simulink model "discrete_system"  (R2022a)
settings: Solver=FixedStepDiscrete  StartTime=0.0  StopTime=10  FixedStep=2E-4
values from neighbouring files (symbols this model uses):
  a1 = -z2/z1    (= 0.769230769231)    [params.m]    (also in params_nolinear_system.m = -z2/z1)
  a2 = z2*eps/z1    (= 2.331002331)    [params.m]    (also in params_nolinear_system.m = z2*eps/z1)
  a3 = z3/z1    (= 2.47815294211)    [params.m]    (also in params_nolinear_system.m = z3/z1)
  a4 = k/z1    (= 1.09686889935)    [params.m]    (also in params_nolinear_system.m = k/z1)
  b1 = -z4/z5    (= 0.822324878959)    [params.m]    (also in params_nolinear_system.m = -z4/z5)
  b2 = z7/(eps*z5)    (= 8.06700706259)    [params.m]    (also in params_nolinear_system.m = z7/(eps*z5))
  b3 = z6/z5    (= 0.963345768584)    [params.m]    (also in params_nolinear_system.m = z6/z5)
  b4 = -k/z5    (= 0.426391767402)    [params.m]    (also in params_nolinear_system.m = -k/z5)
  K = [1 1 1 1]    [params.m]
undefined symbols (not defined in the file or in its folder): DiscIntNeverNeededParam, magnitude
libraries: simulink x2
settings Model: Creator=epyur  LastModifiedBy=epyur
settings SolverCC: ZeroCrossControl=DisableAll  ZeroCrossAlgorithm=Adaptive

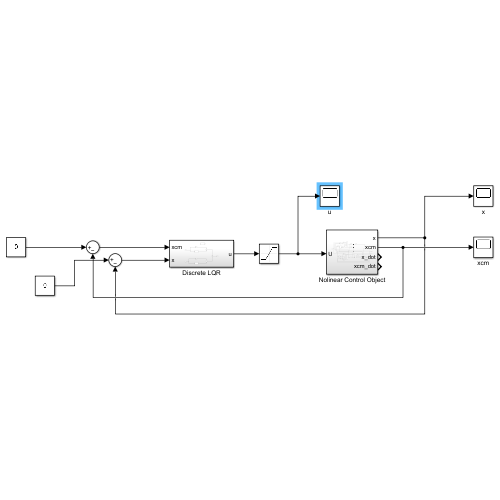
[thumbnail: Simulink's stored preview of the top-level diagram]
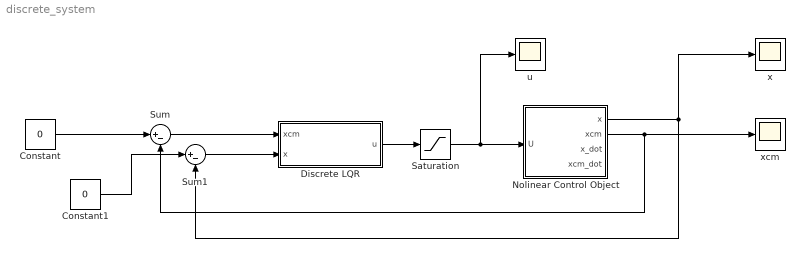
== system discrete_system ==
  Constant : Constant  Value=0
  Constant1 : Constant  Value=0
  Discrete LQR : Subsystem
  Nolinear Control Object : Subsystem
  Saturation : Saturate  UpperLimit=24  LowerLimit=-24
  Sum : Sum  Inputs=|+-
  Sum1 : Sum  Inputs=|+-
  u : Scope
  x : Scope
  xcm : Scope
  wires:
  Saturation/1 -> Nolinear Control Object/1(U), u/1
  Nolinear Control Object/2(xcm) -> Sum/2, xcm/1
  Nolinear Control Object/1(x) -> x/1, Sum1/2
  Discrete LQR/1(u) -> Saturation/1
  Sum/1 -> Discrete LQR/1(xcm)
  Sum1/1 -> Discrete LQR/2(x)
  Constant/1 -> Sum/1
  Constant1/1 -> Sum1/1

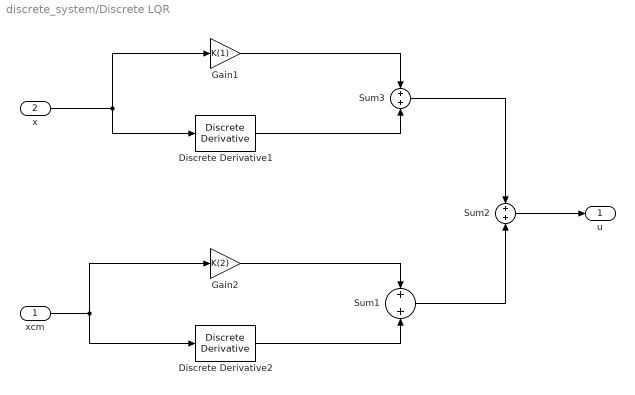
== system discrete_system/Discrete LQR ==
  xcm : Inport
  x : Inport  Port=2
  Discrete Derivative1 : simulink/Discrete/Discrete Derivative  gainval=K(3)  ICPrevScaledInput=0.0  OutMin=[]  OutMax=[]  OutDataType=fixdt(1, 16)  OutScaling=2^-10  DoSatur=off
  Discrete Derivative2 : simulink/Discrete/Discrete Derivative  gainval=K(4)  ICPrevScaledInput=0.0  OutMin=[]  OutMax=[]  OutDataType=fixdt(1, 16)  OutScaling=2^-10  DoSatur=off
  Gain1 : Gain  Gain=K(1)
  Gain2 : Gain  Gain=K(2)
  Sum1 : Sum  Inputs=+|+
  Sum2 : Sum  Inputs=+|+
  Sum3 : Sum  Inputs=+|+
  u : Outport
  wires:
  Sum1/1 -> Sum2/2
  Sum3/1 -> Sum2/1
  Sum2/1 -> u/1
  x/1 -> Discrete Derivative1/1, Gain1/1
  xcm/1 -> Gain2/1, Discrete Derivative2/1
  Discrete Derivative1/1 -> Sum3/2
  Gain1/1 -> Sum3/1
  Discrete Derivative2/1 -> Sum1/2
  Gain2/1 -> Sum1/1

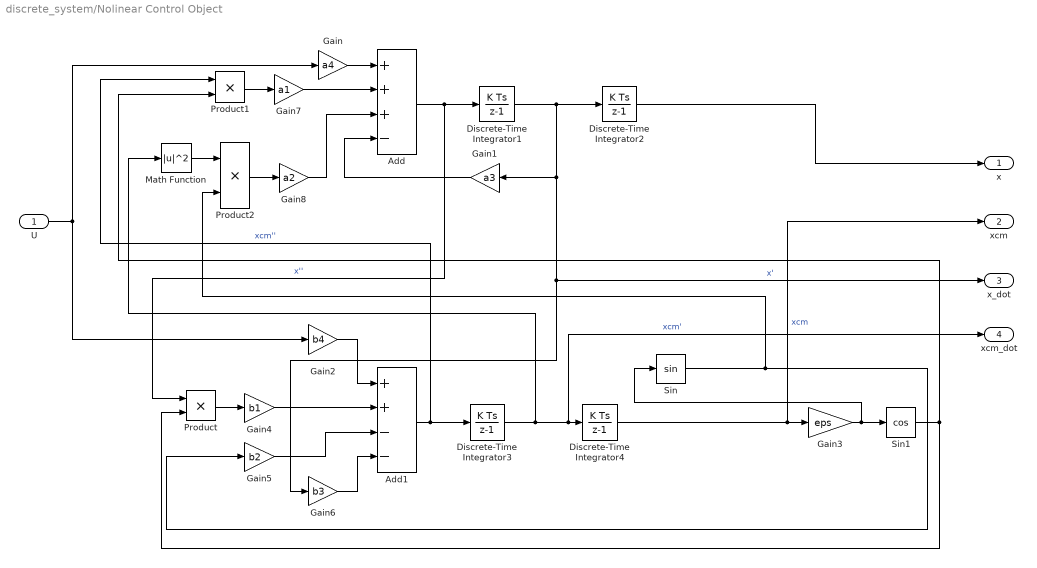
== system discrete_system/Nolinear Control Object ==
  U : Inport
  Add : Sum  Inputs=+++-
  Add1 : Sum  Inputs=++--
  Discrete-Time Integrator1 : DiscreteIntegrator  SampleTime=2e-4  ICPrevOutput=DiscIntNeverNeededParam  ICPrevScaledInput=DiscIntNeverNeededParam
  Discrete-Time Integrator2 : DiscreteIntegrator  SampleTime=2e-4  ICPrevOutput=DiscIntNeverNeededParam  ICPrevScaledInput=DiscIntNeverNeededParam
  Discrete-Time Integrator3 : DiscreteIntegrator  SampleTime=2e-4  ICPrevOutput=DiscIntNeverNeededParam  ICPrevScaledInput=DiscIntNeverNeededParam
  Discrete-Time Integrator4 : DiscreteIntegrator  InitialCondition=-0.144  SampleTime=2e-4  ICPrevOutput=DiscIntNeverNeededParam  ICPrevScaledInput=DiscIntNeverNeededParam
  Gain : Gain  Gain=a4
  Gain1 : Gain  Gain=a3
  Gain2 : Gain  Gain=b4
  Gain3 : Gain  Gain=eps
  Gain4 : Gain  Gain=b1
  Gain5 : Gain  Gain=b2
  Gain6 : Gain  Gain=b3
  Gain7 : Gain  Gain=a1
  Gain8 : Gain  Gain=a2
  Math Function : Math  Operator=magnitude^2
  Product : Product
  Product1 : Product
  Product2 : Product
  Sin : Trigonometry
  Sin1 : Trigonometry  Operator=cos
  x : Outport
  xcm : Outport  Port=2
  x_dot : Outport  Port=3
  xcm_dot : Outport  Port=4
  wires:
  Add/1 -> Discrete-Time Integrator1/1, Product/1  "x''"
  Discrete-Time Integrator1/1 -> Discrete-Time Integrator2/1, Gain6/1, x_dot/1, Gain1/1  "x'"
  Gain/1 -> Add/1
  U/1 -> Gain/1, Gain2/1
  Gain1/1 -> Add/4
  Gain2/1 -> Add1/1
  Add1/1 -> Discrete-Time Integrator3/1, Product1/1  "xcm''"
  Discrete-Time Integrator3/1 -> Math Function/1, Discrete-Time Integrator4/1, xcm_dot/1  "xcm'"
  Discrete-Time Integrator4/1 -> xcm/1, Gain3/1  "xcm"
  Gain3/1 -> Sin/1, Sin1/1
  Gain4/1 -> Add1/2
  Product/1 -> Gain4/1
  Sin1/1 -> Product1/2, Product/2
  Gain5/1 -> Add1/3
  Sin/1 -> Product2/2, Gain5/1
  Gain6/1 -> Add1/4
  Gain7/1 -> Add/2
  Product1/1 -> Gain7/1
  Math Function/1 -> Product2/1
  Product2/1 -> Gain8/1
  Gain8/1 -> Add/3
  Discrete-Time Integrator2/1 -> x/1
